simulink model "Forward_and_inverse_Both"  (R2024b)
settings: Solver=VariableStepAuto  StartTime=0.0  StopTime=7  MaxStep=0.005  RelTol=1e-3
model workspace: external: MATLAB File D:\OneDrive - itc.edu.kh\V4_robot_arm\Import_arm6\Test_Assembly_DataFile.m (data not in the file)
values from neighbouring files (symbols this model uses):
  Reach_max = max(REACH_MAX)    [Workspace_sample.m]
  Reach_min = max(REACH_MIN)    [Workspace_sample.m]
undefined symbols (not defined in the file or in its folder): DiscIntNeverNeededParam, initialPose, maxAngularAcc, maxAngularVel, maxLinearAcc, maxLinearVel, poseTol, smiData, Ts, wps1, X, Y, Z
libraries: sm_lib x140, nesl_utility x52, stmnucleolib x12, simulink x4, vrlib x2, vexcommonlib x2, robotcorelib x2
(part 1 of 6)
settings Model: PacingRate=0.010000  Creator=ASUS  LastModifiedBy=Bro_Chhay
settings OptimizationCC: ReuseModelBlockBuffer=off
settings DebuggingCC: AlgebraicLoopMsg=none  ArtificialAlgebraicLoopMsg=none  InheritedTsInSrcMsg=none
settings RTWCC: GPUComputeCapability=3.5
settings ExplorerConfigSet: InternalSimMechanicsExplorerSettings="<ExplorerConfiguration><canonicalview>default</canonicalview><AnimationSetting><BasePlaybackSpeed>1.0</BasePlaybackSpeed><PlaybackSpeedFactor>1.0</PlaybackSpeedFactor></AnimationSetting><TilePanel><TileInfo><Tiles Columns=\"2\" Count=\"4\" Rows=\"2\"><Column Weight=\"0.5\"/><Column Weight=\"0.5\"/><Row Weight=\"0.5\"/><Row Weight=\"0.5\"/><Tile Height=\"1\" Width=\"1\" X=\"0\" Y=\"0\"/><Tile Height=\"1\" Width=\"1\" X=\"0\" Y=\"1\"/><Tile Height=\"1\" Width=\"1\" X=\"1\" Y=\"0\"/><Tile Height=\"1\" Width=\"1\" X=\"1\" Y=\"1\"/></Tiles></TileInfo><SceneInfo><SceneViewer><BGColor><R>0.800000011920928955</R><G>0.800000011920928955</G><B>0.800000011920928955</B></BGColor><Camera><DoPerspective>off</DoPerspective><Position><X>112.042507163595758</X><Y>-707.89174178180906</Y><Z>378.03229364224967</Z></Position><Center><X>112.042507163595758</X><Y>2.99999040381362647</Y><Z>378.03229364224967</Z></Center><Up><X>0</X><Y>-0</Y><Z>1</Z></Up><ViewLimDist>1</ViewLimDist><YLim>389.373256225585919</YLim><XLim>528.596833306246026</XLim></Camera></SceneViewer><SceneViewer><BGColor><R>0.800000011920928955</R><G>0.800000011920928955</G><B>0.800000011920928955</B></BGColor><Camera><DoPerspective>off</DoPerspective><Position><X>112.042507163595758</X><Y>2.9999928452198219</Y><Z>1115.74949456857576</Z></Position><Center><X>112.042507163595758</X><Y>2.9999928452198219</Y><Z>378.032280824866803</Z></Center><Up><X>0</X><Y>1</Y><Z>-0</Z></Up><ViewLimDist>1</ViewLimDist><YLim>238.200927829742426</YLim><XLim>323.371608420028224</XLim></Camera></SceneViewer><SceneViewer><BGColor><R>0.800000011920928955</R><G>0.800000011920928955</G><B>0.800000011920928955</B></BGColor><Camera><DoPerspective>off</DoPerspective><Position><X>811.571529227276983</X><Y>2.9999928452198219</Y><Z>378.03229364224967</Z></Position><Center><X>112.042497397970806</X><Y>2.9999928452198219</Y><Z>378.03229364224967</Z></Center><Up><X>-0</X><Y>0</Y><Z>1</Z></Up><ViewLimDist>1</ViewLimDist><YLim>389.373256225585919</YLim><XLim>528.596833306246026</XLim></Camera></SceneViewer><SceneViewer><BGColor><R>0.800000011920928955</R><G>0.800000011920928955</G><B>0.800000011920928955</B></BGColor><Camera><DoPerspective>off</DoPerspective><Position><X>445.528454458655347</X><Y>-387.561072008495501</Y><Z>798.922774330656011</Z></Position><Center><X>57.2226628192288871</X><Y>0.744719630931172105</Y><Z>410.616982691205294</Z></Center><Up><X>-0.408248290463863073</X><Y>0.408248290463863073</Y><Z>0.816496580927726145</Z></Up><ViewLimDist>1</ViewLimDist><YLim>413.2447509765625</YLim><XLim>561.003775308298486</XLim></Camera></SceneViewer></SceneInfo></TilePanel><MechEditorPanel><Cameras/><GfxPanelCameraMap/><VideoCreator><PlaybackSpeedRatio>1.0</PlaybackSpeedRatio><FrameRate>60</FrameRate><VideoFormat>MPEG-4</VideoFormat><FrameSize>[1920 1080]</FrameSize></VideoCreator></MechEditorPanel></ExplorerConfiguration>"

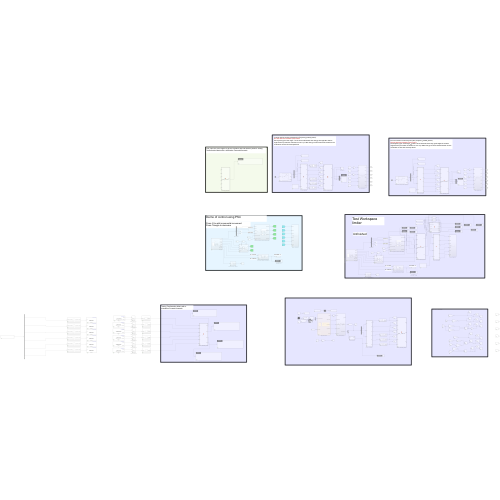
[thumbnail: Simulink's stored preview of the top-level diagram]
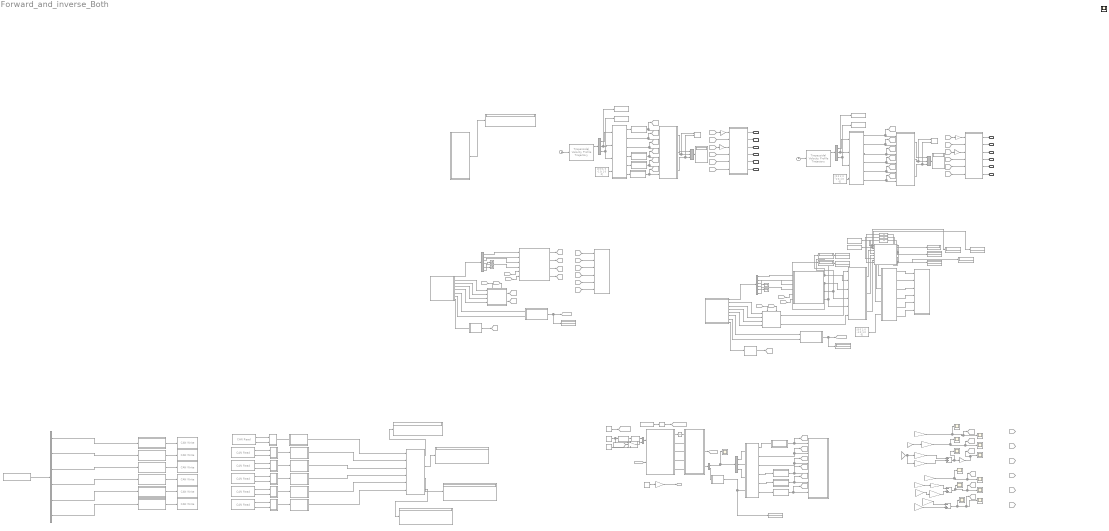
== system Forward_and_inverse_Both ==
  note: First we need to run the trajectory file (Trajectory_matlab_test.m).
      | Give the desired orientation (3x3) matrix.
      | The trajectory give Joint angle $\theta$ to the inverse kinematic then they go throught the relative angle block to prevention of theata run over 2 pi. After that, go to the forward kinematic for the verification as also the simscape block.
  note: cheak after Tranmission
  note: First, input the Joint angles to get the orietaion and end-effector position.Testing Tranformation Matrix with a simlulation Forward Kinematic.
  note: Testing Tranformation Matrix with a simlulation Forward Kinematic
  note: First we need to run the trajectory file (Trajectory_matlab_test.m).
      | Give the desired orientation (3x3) matrix.
      | The trajectory give Joint angle $\theta$ to the inverse kinematic then they go throught the relative angle block to prevention of theata run over 2 pi. After that, go to the forward kinematic for the verification as also the simscape block.
  note: Tri = decrease
  note: O = increase
  note: Initial Delta = 0
  note: Tri = decrease
  note: JoyStick Right
  note: JoyStick Left
  note: O = increase
  note: JoyStick Right
  note: Unfinished
  note: Demo of control using PS4
  note: JoyStick Left
  note: Test Workspace limiter
  note: Press O to add incremental movement
      | Press Triangle to decrease
  note: Initial Delta = 0
  0 ≤ Delta ≤ 0.1 Increment = 0.025 : Display  Commented=on
  0 ≤ Delta ≤ 0.1 Increment = 0.1 : Display  Commented=on
  {1..6} (6 alike) : stmnucleolib/CAN Read  Commented=on  CANModule=1  Identifier=Standard (11-bit identifier)  MsgId=246  MsgLen=8  RemoteFrame=off  OutputStatus=on  SampleTime=-1
      settings: LibrarySourceBlock=stmnucleoh7lib/CAN Read  DataFormat=Raw Data
  6 DOF robot arm : Subsystem  Commented=on
  6 DOF robot arm2 : Subsystem  Commented=on
  Add1 : Sum  Commented=on
  Add2 : Sum  Commented=on  Inputs=-+
  Add3 : Sum  Commented=on  Inputs=-+
  CAN Write : stmnucleolib/CAN Write  Commented=on  CANModule=0  Identifier=Standard (11-bit identifier)  MsgId=1  MsgLen=8  RemoteFrame=off  OutputStatus=off
      settings: LibrarySourceBlock=stmnucleoh7lib/CAN Write  DataFormat=Raw Data
  CAN Write1 : stmnucleolib/CAN Write  Commented=on  CANModule=0  Identifier=Standard (11-bit identifier)  MsgId=2  MsgLen=8  RemoteFrame=off  OutputStatus=off
      settings: LibrarySourceBlock=stmnucleoh7lib/CAN Write  DataFormat=Raw Data
  CAN Write2 : stmnucleolib/CAN Write  Commented=on  CANModule=0  Identifier=Standard (11-bit identifier)  MsgId=3  MsgLen=8  RemoteFrame=off  OutputStatus=off
      settings: LibrarySourceBlock=stmnucleoh7lib/CAN Write  DataFormat=Raw Data
  CAN Write3 : stmnucleolib/CAN Write  Commented=on  CANModule=0  Identifier=Standard (11-bit identifier)  MsgId=4  MsgLen=8  RemoteFrame=off  OutputStatus=off
      settings: LibrarySourceBlock=stmnucleoh7lib/CAN Write  DataFormat=Raw Data
  CAN Write4 : stmnucleolib/CAN Write  Commented=on  CANModule=0  Identifier=Standard (11-bit identifier)  MsgId=5  MsgLen=8  RemoteFrame=off  OutputStatus=off
      settings: LibrarySourceBlock=stmnucleoh7lib/CAN Write  DataFormat=Raw Data
  CAN Write5 : stmnucleolib/CAN Write  Commented=on  CANModule=0  Identifier=Standard (11-bit identifier)  MsgId=6  MsgLen=8  RemoteFrame=off  OutputStatus=off
      settings: LibrarySourceBlock=stmnucleoh7lib/CAN Write  DataFormat=Raw Data
  Clock : Clock  Commented=on
  Clock1 : Clock  Commented=on
  Constant1 : Constant  Commented=on
  Constant11 : Constant  Commented=on  Value=[0 0 1; 0 -1 0; 1 0 0]
  Constant12 : Constant  Commented=on  Value=Reach_max
  Constant13 : Constant  Commented=on  Value=0
  Constant14 : Constant  Commented=on  Value=initialPose
  Constant15 : Constant  Commented=on  Value=Reach_min
  Constant2 : Constant  Commented=on  Value=[0 0 0 0 0 0]
  Constant3 : Constant  Commented=on  Value=[0 0 1; 0 -1 0; 1 0 0]
  Constant4 : Constant  Commented=on  Value=[0 0 1; 0 -1 0; 1 0 0]
  Counter Free-Running : simulink/Sources/Counter Free-Running  Commented=on  NumBits=16  tsamp=-1
  Data Transform1 : Subsystem  Commented=on
  Data Transform2 : Subsystem  Commented=on
  Data Transform3 : Subsystem  Commented=on
  Data Transform4 : Subsystem  Commented=on
  Data Transform5 : Subsystem  Commented=on
  Data Transform6 : Subsystem  Commented=on
  Data Type Conversion : DataTypeConversion  Commented=on  OutDataTypeStr=double  SaturateOnIntegerOverflow=off  RndMeth=Floor
  Demux2 : Demux  Commented=on  Outputs=3
  Demux3 : Demux  Commented=on  Outputs=[3,1]
  Demux5 : Demux  Commented=on  Outputs=3
  Demux6 : Demux  Commented=on  Outputs=3
  Demux8 : Demux  Commented=on  Outputs=6
  Detect Increase : simulink/Logic and Bit Operations/Detect Increase  Commented=on  vinit=0.0  OutDataTypeStr=boolean
  Display{,1..14,17..19} (18 alike) : Display  Commented=on
  Flip the state of a button : Subsystem  Commented=on
  Flip the state of a button1 : Subsystem  Commented=on
  Forward_Kinematic : MATLAB Function  Commented=on  TreatAsAtomicUnit=on
  Forward_Kinematic_Good1 : MATLAB Function  Commented=on  TreatAsAtomicUnit=on
  Forward_Kinematic_Good2 : MATLAB Function  Commented=on  TreatAsAtomicUnit=on
  Forward_Kinematic_Good3 : MATLAB Function  Commented=on  TreatAsAtomicUnit=on
  Forward_Kinematic_Good4 : MATLAB Function  Commented=on  TreatAsAtomicUnit=on
  Forward_Kinematic_Good5 : MATLAB Function  Commented=on  TreatAsAtomicUnit=on
  From{,22..23,38} (4 alike) : From  Commented=on  GotoTag=n
  From1 : From  Commented=on  GotoTag=genPose
  From{10,13,28,36} (4 alike) : From  Commented=on  GotoTag=J5
  From{11,14,29,39} (4 alike) : From  Commented=on  GotoTag=J6
  From{9,12,27,35} (4 alike) : From  Commented=on  GotoTag=J4
  From{15,21,30,37} (4 alike) : From  Commented=on  GotoTag=Delta
  From{2,6,24,32} (4 alike) : From  Commented=on  GotoTag=J1
  From{3,7,25,33} (4 alike) : From  Commented=on  GotoTag=J2
  From{4,8,26,34} (4 alike) : From  Commented=on  GotoTag=J3
  From5 : From  Commented=on  GotoTag=simulation
  Gain{1..2,4,9} (4 alike) : Gain  Commented=on  Gain=32/30
  Gain{10,12,14,16..19} (7 alike) : Gain  Commented=on  Gain=-1
  Gain11 : Gain  Commented=on  Gain=25/15
  Gain13 : Gain  Commented=on  Gain=25/15
  Gain15 : Gain  Commented=on  Gain=Ts  OutDataTypeStr=double
  Gain3 : Gain  Commented=on  Gain=50/16
  Gain5 : Gain  Commented=on  Gain=72/22
  Gain6 : Gain  Commented=on  Gain=48/22
  Gain7 : Gain  Commented=on  Gain=50/36  OutDataTypeStr=Inherit: Same as input
  Gain8 : Gain  Commented=on  Gain=48/22
  Goto{,16,22,38} (4 alike) : Goto  Commented=on  GotoTag=J1
  Goto{1,17,23,37} (4 alike) : Goto  Commented=on  GotoTag=J2
  Goto10 : Goto  Commented=on  GotoTag=q5
  Goto11 : Goto  Commented=on  GotoTag=q6
  Goto12 : Goto  Commented=on  GotoTag=simulation
  Goto13 : Goto  Commented=on  GotoTag=genPose
  Goto14 : Goto  Commented=on  GotoTag=initialPose  TagVisibility=global
  Goto15 : Goto  Commented=on  GotoTag=t  TagVisibility=global
  Goto{2,18,24,39} (4 alike) : Goto  Commented=on  GotoTag=J3
  Goto{3,19,25,40} (4 alike) : Goto  Commented=on  GotoTag=J4
  Goto{4,20,26,41} (4 alike) : Goto  Commented=on  GotoTag=J5
  Goto{5,21,27,43} (4 alike) : Goto  Commented=on  GotoTag=J6
  Goto28 : Goto  Commented=on  GotoTag=Delta
  Goto34 : Goto  Commented=on  GotoTag=n
  Goto36 : Goto  Commented=on  GotoTag=Delta
  Goto42 : Goto  Commented=on  GotoTag=n
  Goto6 : Goto  Commented=on  GotoTag=q1
  Goto7 : Goto  Commented=on  GotoTag=q2
  Goto8 : Goto  Commented=on  GotoTag=q3
  Goto9 : Goto  Commented=on  GotoTag=q4
  Inverse Kinematic : MATLAB Function  Commented=on  TreatAsAtomicUnit=on
  Inverse Kinematic1 : MATLAB Function  Commented=on  TreatAsAtomicUnit=on
  Inverse Kinematic2 : MATLAB Function  Commented=on  TreatAsAtomicUnit=on
  Inverse Kinematic4 : MATLAB Function  Commented=on  TreatAsAtomicUnit=on
  MATLAB Function : MATLAB Function  Commented=on  TreatAsAtomicUnit=on
  Mux : Mux  Commented=on  Inputs=3
  Mux1 : Mux  Commented=on  Inputs=3
  Mux3 : Mux  Commented=on  Inputs=2
  PS4 Demux : Demux  Commented=on  Outputs=6
  PS4 Demux1 : Demux  Commented=on  Outputs=6
  Pulse Generator : DiscretePulseGenerator  Commented=on  PulseType=Time based  Period=30  PulseWidth=5  PhaseDelay=5
  Reshape : Reshape  Commented=on  OutputDimensionality=Column vector (2-D)
  Rotation Matrix : MATLAB Function  Commented=on  TreatAsAtomicUnit=on
  Scope{1,3..14} (13 alike) : Scope  Commented=on
  "Set Delta for the joint movement more Delta, faster the movement" : Subsystem  Commented=on
  "Set Delta for the joint movement more Delta, faster the movement1" : Subsystem  Commented=on
  Set Joint position to where it were left off : Subsystem  Commented=on
  Set Joint position to where it were left off1 : Subsystem  Commented=on
  Simscape Robot1 : Subsystem  Commented=on
  Simscape Robot2 : Subsystem  Commented=on
  Subsystem : Subsystem  Commented=on
      settings: PortSchema="{\"entries\":[{\"content\":{\"sides\":[{\"content\":{\"connectorIds\":[\"In1\",\"In2\",\"In3\",\"In4\"]},\"type\":\"ConnectorPlacement.EquallySpacedRectSide\",\"uuid\":\"934df258-a69f-45fc-920e-d96d4c7e69c4\"},{\"content\":{\"connectorIds\":[\"Out1\",\"Out2\"],\"side\":\"RIGHT\"},\"type\":\"ConnectorPlacement.EquallySpacedRectSide\",\"uuid\":\"4248c0a4-0efa-4e68-894f-9df7c5b1e3ab\"},{\"content\":{\"connectorIds\":[\"In5\",\"In6\"],\"side\":\"TOP\"},\"type\":\"ConnectorPlacement.EquallySpacedRectSide\",\"uuid\":\"db1bee13-57d6-4361-8657-1365417e1e26\"}]},\"type\":\"ConnectorPlacement.EquallySpacedConnector\",\"uuid\":\"c32f6b1b-3465-4573-ab20-ef0ae83e0fed\"}],\"packageUris\":[\"http://schema.mathworks.com/mf0/Connector/R2020b\"],\"version\":\"1.0\"}"
  Subsystem1 : Subsystem  Commented=on
  Subsystem10 : Subsystem  Commented=on
  Subsystem11 : Subsystem  Commented=on
  Subsystem12 : Subsystem  Commented=on
  Subsystem13 : Subsystem  Commented=on
  Subsystem14 : Subsystem  Commented=on
  Subsystem15 : Subsystem  Commented=on
  Subsystem16 : Subsystem  Commented=on
  Subsystem17 : Subsystem  Commented=on
  Subsystem18 : Subsystem  Commented=on
  Subsystem19 : Subsystem  Commented=on
  Subsystem2 : Subsystem  Commented=on
  Subsystem20 : Subsystem  Commented=on
      settings: PortSchema="{\"entries\":[{\"content\":{\"sides\":[{\"content\":{\"connectorIds\":[\"In1\",\"In2\",\"In3\",\"In4\"]},\"type\":\"ConnectorPlacement.EquallySpacedRectSide\",\"uuid\":\"934df258-a69f-45fc-920e-d96d4c7e69c4\"},{\"content\":{\"connectorIds\":[\"Out1\",\"Out2\"],\"side\":\"RIGHT\"},\"type\":\"ConnectorPlacement.EquallySpacedRectSide\",\"uuid\":\"4248c0a4-0efa-4e68-894f-9df7c5b1e3ab\"},{\"content\":{\"connectorIds\":[\"In5\",\"In6\"],\"side\":\"TOP\"},\"type\":\"ConnectorPlacement.EquallySpacedRectSide\",\"uuid\":\"db1bee13-57d6-4361-8657-1365417e1e26\"}]},\"type\":\"ConnectorPlacement.EquallySpacedConnector\",\"uuid\":\"c32f6b1b-3465-4573-ab20-ef0ae83e0fed\"}],\"packageUris\":[\"http://schema.mathworks.com/mf0/Connector/R2020b\"],\"version\":\"1.0\"}"
  Subsystem21 : Subsystem  Commented=on
  Subsystem24 : Subsystem  Commented=on
  Subsystem25 : Subsystem  Commented=on
  Subsystem3 : Subsystem  Commented=on
  Subsystem4 : Subsystem  Commented=on
  Subsystem5 : Subsystem  Commented=on
  Subsystem6 : Subsystem  Commented=on
  Subsystem7 : Subsystem  Commented=on
  Subsystem8 : Subsystem  Commented=on
  Subsystem9 : Subsystem  Commented=on
  Switch4 : Switch  Commented=on  Criteria=u2 > Threshold  SaturateOnIntegerOverflow=off  InputSameDT=off
  Terminator{,1..3} (4 alike) : Terminator  Commented=on
  To Workspace : ToWorkspace  Commented=on  VariableName=Yin  SampleTime=-1
      settings: Save2DSignal=2-D array (concatenate along first dimension)
  To Workspace1 : ToWorkspace  Commented=on  VariableName=Zin1  SampleTime=-1
      settings: Save2DSignal=2-D array (concatenate along first dimension)
  To Workspace2 : ToWorkspace  Commented=on  VariableName=Yin1  SampleTime=-1
      settings: Save2DSignal=2-D array (concatenate along first dimension)
  To Workspace3 : ToWorkspace  Commented=on  VariableName=Zin  SampleTime=-1
      settings: Save2DSignal=2-D array (concatenate along first dimension)
  Trapezoidal Velocity Profile Trajectory : robotcorelib/Trapezoidal Velocity Profile Trajectory  Commented=on  WaypointSource=Internal  Waypoints=waypoints_6  NumParams=1  Parameter1=End Time  Parameter2=End Time  ParameterSource=Internal  PeakVelocity=[ 2; 2 ]  Acceleration=[ 1; 2 ]  EndTime=2  AccelTime=[ 1; 2 ]  SimulateUsing=Interpreted execution
  Trapezoidal Velocity Profile Trajectory1 : robotcorelib/Trapezoidal Velocity Profile Trajectory  Commented=on  WaypointSource=Internal  Waypoints=Way4  NumParams=1  Parameter1=End Time  Parameter2=End Time  ParameterSource=Internal  PeakVelocity=[ 2; 2 ]  Acceleration=[ 1; 2 ]  EndTime=2  AccelTime=[ 1; 2 ]  SimulateUsing=Interpreted execution
  Unit Delay{,1..3} (4 alike) : UnitDelay  Commented=on  SampleTime=-1  HasFrameUpgradeWarning=on
  Waypoint Planner : Stateflow chart  Commented=on  TreatAsAtomicUnit=on
      settings: PortSchema="{\"entries\":[{\"content\":{\"sides\":[{\"content\":{\"connectorIds\":[\"In2\",\"In1\"]},\"type\":\"ConnectorPlacement.EquallySpacedRectSide\",\"uuid\":\"2f7816bf-e041-4d80-a35c-f5abf025ca4f\"},{\"content\":{\"connectorIds\":[\"Out5\",\"Out1\",\"Out2\",\"Out3\",\"Out4\"],\"side\":\"RIGHT\"},\"type\":\"ConnectorPlacement.EquallySpacedRectSide\",\"uuid\":\"030a9877-c717-421f-9736-0adf27f6f35f\"},{\"content\":{\"side\":\"TOP\"},\"type\":\"ConnectorPlacement.EquallySpacedRectSide\",\"uuid\":\"ba023d22-bb45-4b84-a72f-1110f01393be\"}]},\"type\":\"ConnectorPlacement.EquallySpacedConnector\",\"uuid\":\"d2a85391-dfa2-4741-8917-4ca0c8ef44a5\"}],\"packageUris\":[\"http://schema.mathworks.com/mf0/Connector/R2020b\"],\"version\":\"1.0\"}"
  Waypoint Trajectory : Subsystem  Commented=on
  XY Graph1 : Record  Commented=on  VariableName=recordout2  RecordToWorkspace=on  FileSettingsInternal="{\"entries\":[{\"content\":{\"excelSettings\":{\"content\":{},\"type\":\"Streamout.ExcelSettings\"}},\"type\":\"Streamout.FileSettingStorage\",\"uuid\":\"\"}],\"packageUris\":[\"http:\\/\\/schema.mathworks.com\\/mf0\\/streamout_blocks\\/R2020a\"],\"version\":\"1.0\"}"  Layout=[1 1]  SignalsInternal="{\"entries\":[{\"content\":{},\"type\":\"RecordBlkView.InputSignals\",\"uuid\":\"\"}],\"packageUris\":[\"http:\\/\\/schema.mathworks.com\\/mf0\\/streamout_blocks\\/R2020a\"],\"version\":\"1.0\"}"  VisualizationBindings="{\"xyplotplugin\":{\"info\":[{\"series\":[],\"subplotID\":1}]}}"  CompatibilityTag=XY
  XY Graph2 : Record  Commented=on  VariableName=recordout2  RecordToWorkspace=on  FileSettingsInternal="{\"entries\":[{\"content\":{\"excelSettings\":{\"content\":{},\"type\":\"Streamout.ExcelSettings\"}},\"type\":\"Streamout.FileSettingStorage\",\"uuid\":\"\"}],\"packageUris\":[\"http:\\/\\/schema.mathworks.com\\/mf0\\/streamout_blocks\\/R2020a\"],\"version\":\"1.0\"}"  Layout=[1 1]  SignalsInternal="{\"entries\":[{\"content\":{\"signals\":[{\"content\":{\"blockPath\":[],\"dimensions\":[1],\"domain\":\"\",\"lineColor\":\"#a2142f\",\"plots\":[ 1 ],\"port\":1,\"signalID\":1,\"signalName\":\"Forward_Kinematic_Good4:2\"},\"type\":\"RecordBlkView.Signal\",\"uuid\":\"\"},{\"content\":{\"blockPath\":[],\"dimensions\":[1],\"domain\":\"\",\"lineColor\":\"#139fff\",\"plots\":[ 1 ],\"port\":2,\"signalID\":2,\"signalName\":\"Forward_Kinematic_Good4:3\"},\"type\":\"RecordBlkView.Signal\",\"uuid\":\"\"}]},\"type\":\"RecordBlkView.InputSignals\",\"uuid\":\"\"}],\"packageUris\":[\"http:\\/\\/schema.mathworks.com\\/mf0\\/streamout_blocks\\/R2020a\"],\"version\":\"1.0\"}"  VisualizationBindings="{\"xyplotplugin\":{\"info\":[{\"series\":[{\"bindingParametersList\":[{\"parameter\":\"X-Axis\",\"signalID\":1,\"signalName\":\"Forward_Kinematic_Good4:2\"},{\"parameter\":\"Y-Axis\",\"signalID\":2,\"signalName\":\"Forward_Kinematic_Good4:3\"}],\"seriesID\":0}],\"subplotID\":1}]}}"  CompatibilityTag=XY
  Output : Outport
  Output1 : Outport  Port=2
  Output2 : Outport  Port=3
  Output3 : Outport  Port=4
  Output4 : Outport  Port=5
  Output5 : Outport  Port=6
  Output6 : Outport  Port=7
  Output7 : Outport  Port=8
  Output8 : Outport  Port=9
  Output9 : Outport  Port=10
  Output10 : Outport  Port=11
  Output11 : Outport  Port=12
  Scope2 : Scope
  wires:
  Forward_Kinematic_Good2/4(R36) -> Display18/1
  Forward_Kinematic_Good2/3(R03) -> Display17/1
  Forward_Kinematic_Good2/2(R06) -> Display10/1
  Constant2/1 -> Demux8/1
  Forward_Kinematic_Good2/1(A06) -> Display19/1
  Demux8/3 -> Subsystem2/1(Desired Position)
  Subsystem1/1(Output to CAN) -> CAN Write1/1
  Demux8/1 -> Subsystem4/1(Desired Position)
  Subsystem5/1(Output to CAN) -> CAN Write4/1
  Subsystem6/1(Output to CAN) -> CAN Write5/1
  Demux8/5 -> Subsystem5/1(Desired Position)
  Demux8/6 -> Subsystem6/1(Desired Position)
  Subsystem2/1(Output to CAN) -> CAN Write2/1
  Subsystem4/1(Output to CAN) -> CAN Write/1
  Demux8/2 -> Subsystem1/1(Desired Position)
  Demux8/4 -> Subsystem3/1(Desired Position)
  Subsystem3/1(Output to CAN) -> CAN Write3/1
  Data Transform2/1(Data_T) -> Subsystem8/1(data)
  Subsystem7/1(position) -> Forward_Kinematic_Good2/1(th1)
  Data Transform3/1(Data_T) -> Subsystem9/1(data)
  Subsystem11/1(position) -> Forward_Kinematic_Good2/5(th5)
  Subsystem12/1(position) -> Forward_Kinematic_Good2/6(th6)
  Subsystem10/1(position) -> Forward_Kinematic_Good2/4(th4)
  Data Transform5/1(Data_T) -> Subsystem11/1(data)
  Subsystem8/1(position) -> Forward_Kinematic_Good2/2(th2)
  1/2 -> Data Transform2/2(In2)
  6/1 -> Data Transform6/1(In1)
  6/2 -> Data Transform6/2(In2)
  2/2 -> Data Transform3/2(In2)
  Data Transform1/1(Data_T) -> Subsystem7/1(data)
  5/1 -> Data Transform5/1(In1)
  4/2 -> Data Transform4/2(In2)
  Data Transform6/1(Data_T) -> Subsystem12/1(data)
  3/2 -> Data Transform1/2(In2)
  Data Transform4/1(Data_T) -> Subsystem10/1(data)
  2/1 -> Data Transform3/1(In1)
  3/1 -> Data Transform1/1(In1)
  4/1 -> Data Transform4/1(In1)
  1/1 -> Data Transform2/1(In1)
  5/2 -> Data Transform5/2(In2)
  Subsystem9/1(position) -> Forward_Kinematic_Good2/3(th3)
  Gain3/1 -> Scope6/1, Scope12/1, Goto9/1  "J4"
  Gain5/1 -> Scope10/1, Goto7/1, Scope4/1  "J2"
  Gain1/1 -> Add2/1
  Gain8/1 -> Add1/2
  Add1/1 -> Gain12/1, Scope5/1  "J3"
  Gain4/1 -> Add3/2
  Gain6/1 -> Add1/1
  Gain13/1 -> Gain9/1
  Gain7/1 -> Scope3/1, Scope9/1, Goto6/1  "J1"
  Add2/1 -> Scope7/1, Scope13/1, Goto10/1  "J5"
  Gain11/1 -> Gain1/1
  Add3/1 -> Scope8/1, Scope14/1, Goto11/1  "J6"
  Gain9/1 -> Add2/2
  Trapezoidal Velocity Profile Trajectory/1 -> Demux6/1
  Gain12/1 -> Scope11/1, Goto8/1
  Gain2/1 -> Add3/1
  Gain10/1 -> Gain5/1
  Gain14/1 -> Gain8/1, Gain6/1
  Constant13/1 -> Switch4/3
  Waypoint Trajectory/2(genPose) -> Goto13/1
  Demux3/2 -> Rotation Matrix/1(roll)
  Waypoint Planner/3(targetPose) -> Waypoint Trajectory/4(targetPose)
  Waypoint Trajectory/3(filteredPose) -> Demux3/1
  Switch4/1 -> Mux3/2
  Mux3/1 -> Waypoint Planner/2(semiAutoButton)
  Waypoint Planner/1(departTime) -> Waypoint Trajectory/2(departTime)
  From1/1 -> Waypoint Planner/1(genPose)
  Detect Increase/1 -> Data Type Conversion/1
  Pulse Generator/1 -> Switch4/1, Detect Increase/1
  Unit Delay/1 -> Waypoint Trajectory/1(mode)
  Waypoint Planner/4(maxVel) -> Waypoint Trajectory/5(maxVel)
  Demux3/1 -> Demux5/1, Scope1/1
  Counter Free-Running/1 -> Gain15/1
  Reshape/1 -> Goto14/1
  Rotation Matrix/1(R06) -> Display/1, Inverse Kinematic1/4(R06)
  Waypoint Planner/2(departPose) -> Waypoint Trajectory/3(departPose)
  Gain15/1 -> Goto15/1
  Constant1/1 -> Goto12/1
  Data Type Conversion/1 -> Mux3/1
  Constant14/1 -> Reshape/1
  From5/1 -> Switch4/2
  Waypoint Planner/5(mode) -> Unit Delay/1
  Subsystem16/1(angle) -> Forward_Kinematic_Good3/5(th5), Goto4/1
  Subsystem17/1(angle) -> Forward_Kinematic_Good3/6(th6), Goto5/1
  Inverse Kinematic1/4(q4) -> Subsystem15/1(q1)
  Inverse Kinematic1/1(q1) -> Subsystem13/1(q1)
  Inverse Kinematic1/6(q6) -> Subsystem17/1(q1)  "q6"
  Inverse Kinematic1/3(q3) -> Goto2/1, Forward_Kinematic_Good3/3(th3)  "q3"
  Inverse Kinematic1/5(q5) -> Subsystem16/1(q1)
  Subsystem13/1(angle) -> Forward_Kinematic_Good3/1(th1), Goto/1
  Inverse Kinematic1/2(q2) -> Forward_Kinematic_Good3/2(th2), Goto1/1  "q2"
  Subsystem15/1(angle) -> Forward_Kinematic_Good3/4(th4), Goto3/1
  Demux5/1 -> Inverse Kinematic1/1(Px)
  Demux5/2 -> Inverse Kinematic1/2(Py)
  Demux5/3 -> Inverse Kinematic1/3(Pz)
  Subsystem14/1(angle) -> Forward_Kinematic_Good1/1(th1), Goto16/1
  Inverse Kinematic/4(q4) -> Subsystem18/1(q1)
  Demux6/2 -> To Workspace/1, Inverse Kinematic/2(Py)
  Inverse Kinematic/3(q3) -> Forward_Kinematic_Good1/3(th3), Goto18/1  "q3"
  Demux6/3 -> To Workspace1/1, Inverse Kinematic/3(Pz)
  Subsystem25/1(angle) -> Forward_Kinematic_Good1/6(th6), Goto21/1
  Inverse Kinematic/2(q2) -> Forward_Kinematic_Good1/2(th2), Goto17/1  "q2"
  Inverse Kinematic/6(q6) -> Subsystem25/1(q1)  "q6"
  Inverse Kinematic/5(q5) -> Subsystem24/1(q1)
  Inverse Kinematic/1(q1) -> Subsystem14/1(q1)
  Demux6/1 -> Inverse Kinematic/1(Px)
  Subsystem18/1(angle) -> Forward_Kinematic_Good1/4(th4), Goto19/1
  Constant3/1 -> Inverse Kinematic/4(R06)
  Subsystem24/1(angle) -> Forward_Kinematic_Good1/5(th5), Goto20/1
  Forward_Kinematic_Good1/2(Py) -> XY Graph1/1, Mux/2
  Forward_Kinematic_Good1/3(Pz) -> Mux/3, XY Graph1/2
  Forward_Kinematic_Good1/1(Px) -> Mux/1
  Mux/1 -> Display2/1
  Clock/1 -> Trapezoidal Velocity Profile Trajectory/1
  From24/1 -> Gain18/1
  From25/1 -> Simscape Robot1/2(q2)
  Gain16/1 -> Simscape Robot1/3(q3)
  Gain18/1 -> Simscape Robot1/1(q1)
  From27/1 -> Simscape Robot1/4(q4)
  From26/1 -> Gain16/1
  From29/1 -> Simscape Robot1/6(q6)
  From28/1 -> Simscape Robot1/5(q5)
  Simscape Robot1/1(qm1) -> Output/1
  Simscape Robot1/2(qm2) -> Output1/1
  Simscape Robot1/3(qm3) -> Output2/1
  Simscape Robot1/4(qm4) -> Output3/1
  Simscape Robot1/5(qm5) -> Output4/1
  Simscape Robot1/6(qm6) -> Output5/1
  Simscape Robot2/2(qm2) -> Output7/1
  Simscape Robot2/3(qm3) -> Output8/1
  Simscape Robot2/6(qm6) -> Output11/1
  Simscape Robot2/5(qm5) -> Output10/1
  Gain19/1 -> Simscape Robot2/1(q1)
  From3/1 -> Simscape Robot2/2(q2)
  Simscape Robot2/4(qm4) -> Output9/1
  From13/1 -> Simscape Robot2/5(q5)
  Inverse Kinematic2/4(q4) -> Forward_Kinematic_Good4/4(th4), Goto25/1
  Inverse Kinematic2/3(q3) -> Goto24/1, Forward_Kinematic_Good4/3(th3)  "q3"
  Demux2/2 -> To Workspace2/1, Inverse Kinematic2/2(Py)
  Forward_Kinematic_Good4/2(Py) -> XY Graph2/1, Mux1/2
  From14/1 -> Simscape Robot2/6(q6)
  Forward_Kinematic_Good4/3(Pz) -> Mux1/3, XY Graph2/2
  Inverse Kinematic2/6(q6) -> Forward_Kinematic_Good4/6(th6), Goto27/1  "q6"
  Inverse Kinematic2/1(q1) -> Forward_Kinematic_Good4/1(th1), Goto22/1
  Inverse Kinematic2/5(q5) -> Forward_Kinematic_Good4/5(th5), Goto26/1
  Forward_Kinematic_Good4/1(Px) -> Mux1/1
  Clock1/1 -> Trapezoidal Velocity Profile Trajectory1/1
  Demux2/1 -> Inverse Kinematic2/1(Px)
  Constant4/1 -> Inverse Kinematic2/4(R06)
  Demux2/3 -> To Workspace3/1, Inverse Kinematic2/3(Pz)
  From2/1 -> Gain19/1
  Mux1/1 -> Display1/1
  Trapezoidal Velocity Profile Trajectory1/1 -> Demux2/1
  Inverse Kinematic2/2(q2) -> Forward_Kinematic_Good4/2(th2), Goto23/1  "q2"
  From4/1 -> Gain17/1
  Gain17/1 -> Simscape Robot2/3(q3)
  Simscape Robot2/1(qm1) -> Output6/1
  From12/1 -> Simscape Robot2/4(q4)
  Forward_Kinematic/1(A0_6) -> Display4/1
  From36/1 -> 6 DOF robot arm2/5(joint5)
  PS4 Demux1/3 -> Set Joint position to where it were left off1/3(pos2)
  Subsystem21/6(D8_left) -> "Set Delta for the joint movement more Delta, faster the movement1"/1(O)
  Set Joint position to where it were left off1/1(posfinal2) -> Goto37/1
  Subsystem21/1(Out1) -> PS4 Demux1/1
  From15/1 -> Set Joint position to where it were left off/5(pos incremental)
  From22/1 -> Subsystem/6(n)
  Constant15/1 -> Display8/1, MATLAB Function/1(Reach_min)
  Set Joint position to where it were left off1/4(posfinal5) -> Goto41/1
  Inverse Kinematic4/4(q4) -> 6 DOF robot arm/4(joint4)
  Subsystem19/7(D8_down) -> "Set Delta for the joint movement more Delta, faster the movement"/2(Tri)
  From23/1 -> Set Joint position to where it were left off1/6(coeff to set pos 0)
  MATLAB Function/1(x_out) -> Unit Delay2/1, Inverse Kinematic4/1(Px), Display3/1
  From37/1 -> Subsystem20/5(delta)
  Subsystem21/2(D5_up) -> Subsystem20/1(L1)
  Subsystem21/4(D_right) -> Subsystem20/3(Dpad R)
  PS4 Demux1/1 -> Set Joint position to where it were left off1/1(pos1)
  Subsystem19/8(D8_right) -> Flip the state of a button/1(X)
  From/1 -> Set Joint position to where it were left off/6(coeff to set pos 0)
  Subsystem21/3(D6_up) -> Subsystem20/2(R1)
  From21/1 -> Subsystem/5(delta)
  Flip the state of a button1/1(n_out) -> Goto42/1
  Subsystem21/8(D8_right) -> Flip the state of a button1/1(X)
  Subsystem19/1(Out1) -> PS4 Demux/1
  From39/1 -> 6 DOF robot arm2/6(joint6)
  PS4 Demux/1 -> Set Joint position to where it were left off/1(pos1)
  Set Joint position to where it were left off/2(posfinal3) -> Display12/1, Forward_Kinematic_Good5/3(th3)
  Subsystem19/5(D_left) -> Subsystem/4(Dpad L)
  Unit Delay2/1 -> MATLAB Function/4(x_error)
  From33/1 -> 6 DOF robot arm2/2(joint2)
  PS4 Demux1/6 -> Set Joint position to where it were left off1/4(pos4)
  Constant11/1 -> Inverse Kinematic4/4(R06)
  Inverse Kinematic4/6(q6) -> 6 DOF robot arm/6(joint6)  "q6"
  Forward_Kinematic_Good5/3(Pz) -> MATLAB Function/7(z)
  Set Joint position to where it were left off/1(posfinal2) -> Display11/1, Forward_Kinematic_Good5/2(th2)
  Subsystem20/2(J6) -> Goto43/1
  "Set Delta for the joint movement more Delta, faster the movement"/1(Output) -> 0 ≤ Delta ≤ 0.1 Increment = 0.025/1, Goto28/1
  PS4 Demux1/4 -> Terminator2/1
  Subsystem/2(J6) -> Forward_Kinematic_Good5/6(th6)
  Unit Delay1/1 -> MATLAB Function/6(y_error)
  Inverse Kinematic4/2(q2) -> 6 DOF robot arm/2(joint2)  "q2"
  Subsystem19/2(D5_up) -> Subsystem/1(L1)
  Subsystem21/5(D_left) -> Subsystem20/4(Dpad L)
  PS4 Demux/6 -> Set Joint position to where it were left off/4(pos4)
  PS4 Demux/2 -> Set Joint position to where it were left off/2(pos3)
  From34/1 -> 6 DOF robot arm2/3(joint3)
  Set Joint position to where it were left off1/3(posfinal4) -> Goto40/1
  "Set Delta for the joint movement more Delta, faster the movement1"/1(Output) -> 0 ≤ Delta ≤ 0.1 Increment = 0.1/1, Goto36/1
  From38/1 -> Subsystem20/6(n)
  Set Joint position to where it were left off/4(posfinal5) -> Display14/1, Forward_Kinematic_Good5/5(th5)
  From32/1 -> 6 DOF robot arm2/1(joint1)
  Set Joint position to where it were left off/3(posfinal4) -> Display13/1, Forward_Kinematic_Good5/4(th4)
  PS4 Demux1/2 -> Set Joint position to where it were left off1/2(pos3)
  Inverse Kinematic4/1(q1) -> 6 DOF robot arm/1(joint1)
  From35/1 -> 6 DOF robot arm2/4(joint4)
  Inverse Kinematic4/3(q3) -> 6 DOF robot arm/3(joint3)  "q3"
  Forward_Kinematic_Good5/2(Py) -> MATLAB Function/5(y)
  Subsystem21/7(D8_down) -> "Set Delta for the joint movement more Delta, faster the movement1"/2(Tri)
  Forward_Kinematic_Good5/1(Px) -> MATLAB Function/3(x)
  From30/1 -> Set Joint position to where it were left off1/5(pos incremental)
  Subsystem19/3(D6_up) -> Subsystem/2(R1)
  Flip the state of a button/1(n_out) -> Goto34/1
  Subsystem20/1(J1) -> Goto38/1
  Constant12/1 -> Display9/1, MATLAB Function/2(Reach_max)
  Subsystem19/6(D8_left) -> "Set Delta for the joint movement more Delta, faster the movement"/1(O)
  Subsystem19/4(D_right) -> Subsystem/3(Dpad R)
  PS4 Demux/4 -> Terminator/1
  PS4 Demux/3 -> Set Joint position to where it were left off/3(pos2)
  PS4 Demux1/5 -> Terminator3/1
  Subsystem/1(J1) -> Forward_Kinematic_Good5/1(th1)
  MATLAB Function/4(Out) -> Display7/1
  MATLAB Function/3(z_out) -> Display6/1, Unit Delay3/1, Inverse Kinematic4/3(Pz)
  Unit Delay3/1 -> MATLAB Function/8(z_error)
  MATLAB Function/2(y_out) -> Unit Delay1/1, Inverse Kinematic4/2(Py), Display5/1
  PS4 Demux/5 -> Terminator1/1
  Set Joint position to where it were left off1/2(posfinal3) -> Goto39/1
  Inverse Kinematic4/5(q5) -> 6 DOF robot arm/5(joint5)

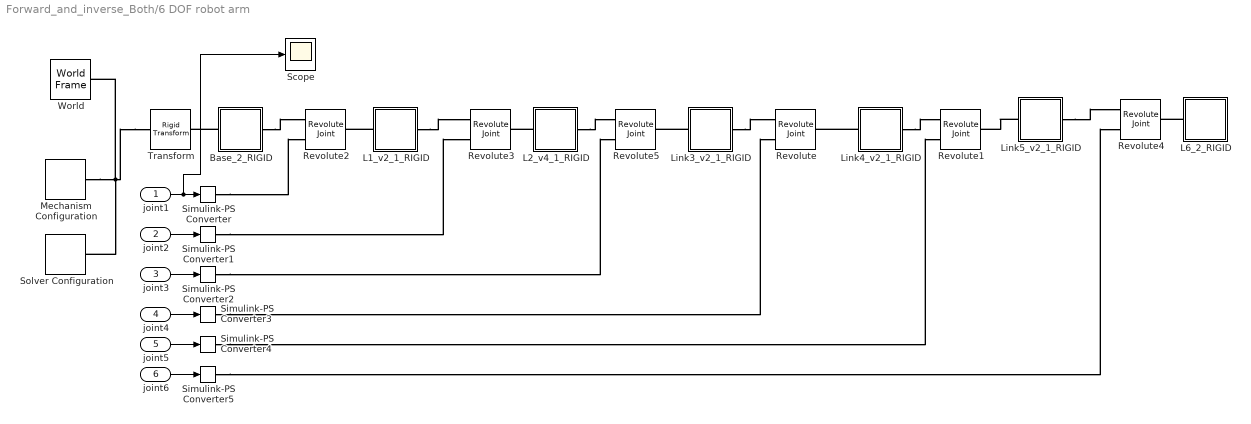
== system Forward_and_inverse_Both/6 DOF robot arm ==
  joint1 : Inport
  joint2 : Inport  Port=2
  joint3 : Inport  Port=3
  joint4 : Inport  Port=4
  joint5 : Inport  Port=5
  joint6 : Inport  Port=6
  Base_2_RIGID : Subsystem
  L1_v2_1_RIGID : Subsystem
  L2_v4_1_RIGID : Subsystem
  L6_2_RIGID : Subsystem
  Link3_v2_1_RIGID : Subsystem
  Link4_v2_1_RIGID : Subsystem
  Link5_v2_1_RIGID : Subsystem
  Mechanism Configuration : sm_lib/Utilities/Mechanism Configuration  UniformGravity=Constant  GravityVector=[0 0 -9.80665]  GravityVectorUnits=m/s^2  LinearizationDelta=0.001  JointModeTransitionNonlinearIterations=2
  Revolute : sm_lib/Joints/Revolute Joint  JointMode=Normal  CompositeWrenchDir=FollowerOnBase  CompositeWrenchFrame=BaseFrame  SenseConstraintForce=off  SenseConstraintTorque=off  SenseTotalForce=off  SenseTotalTorque=off  PositionTargetSpecify=off  PositionTargetPriority=Low  PositionTargetValue=smiData.RevoluteJoint(1).Rz.Pos  PositionTargetValueUnits=deg  VelocityTargetSpecify=off  VelocityTargetPriority=High  VelocityTargetValue=0  VelocityTargetValueUnits=deg/s  EquilibriumPosition=0  EquilibriumPositionUnits=deg  SpringStiffness=0  SpringStiffnessUnits=N*m/deg  DampingCoefficient=0  DampingCoefficientUnits=N*m/(deg/s)  LowerLimitSpecify=off  LowerLimitBound=-90  LowerLimitBoundUnits=deg  LowerLimitStiffness=1e4  LowerLimitStiffnessUnits=N*m/deg  LowerLimitDamping=10  LowerLimitDampingUnits=N*m/(deg/s)  LowerLimitTransitionRegionWidth=0.1  LowerLimitTransitionRegionWidthUnits=deg  UpperLimitSpecify=off  UpperLimitBound=90  UpperLimitBoundUnits=deg  UpperLimitStiffness=1e4  UpperLimitStiffnessUnits=N*m/deg  UpperLimitDamping=10  UpperLimitDampingUnits=N*m/(deg/s)  UpperLimitTransitionRegionWidth=0.1  UpperLimitTransitionRegionWidthUnits=deg  TorqueActuationMode=ComputedTorque  MotionActuationMode=InputMotion  SensePosition=off  SenseVelocity=off  SenseAcceleration=off  SenseTorqueForce=off  SenseLowerLimitTorqueForce=off  SenseUpperLimitTorqueForce=off
  Revolute1 : sm_lib/Joints/Revolute Joint  JointMode=Normal  CompositeWrenchDir=FollowerOnBase  CompositeWrenchFrame=BaseFrame  SenseConstraintForce=off  SenseConstraintTorque=off  SenseTotalForce=off  SenseTotalTorque=off  PositionTargetSpecify=off  PositionTargetPriority=Low  PositionTargetValue=smiData.RevoluteJoint(2).Rz.Pos  PositionTargetValueUnits=deg  VelocityTargetSpecify=off  VelocityTargetPriority=High  VelocityTargetValue=0  VelocityTargetValueUnits=deg/s  EquilibriumPosition=0  EquilibriumPositionUnits=deg  SpringStiffness=0  SpringStiffnessUnits=N*m/deg  DampingCoefficient=0  DampingCoefficientUnits=N*m/(deg/s)  LowerLimitSpecify=off  LowerLimitBound=-90  LowerLimitBoundUnits=deg  LowerLimitStiffness=1e4  LowerLimitStiffnessUnits=N*m/deg  LowerLimitDamping=10  LowerLimitDampingUnits=N*m/(deg/s)  LowerLimitTransitionRegionWidth=0.1  LowerLimitTransitionRegionWidthUnits=deg  UpperLimitSpecify=off  UpperLimitBound=90  UpperLimitBoundUnits=deg  UpperLimitStiffness=1e4  UpperLimitStiffnessUnits=N*m/deg  UpperLimitDamping=10  UpperLimitDampingUnits=N*m/(deg/s)  UpperLimitTransitionRegionWidth=0.1  UpperLimitTransitionRegionWidthUnits=deg  TorqueActuationMode=ComputedTorque  MotionActuationMode=InputMotion  SensePosition=off  SenseVelocity=off  SenseAcceleration=off  SenseTorqueForce=off  SenseLowerLimitTorqueForce=off  SenseUpperLimitTorqueForce=off
  Revolute2 : sm_lib/Joints/Revolute Joint  JointMode=Normal  CompositeWrenchDir=FollowerOnBase  CompositeWrenchFrame=BaseFrame  SenseConstraintForce=off  SenseConstraintTorque=off  SenseTotalForce=off  SenseTotalTorque=off  PositionTargetSpecify=off  PositionTargetPriority=Low  PositionTargetValue=smiData.RevoluteJoint(3).Rz.Pos  PositionTargetValueUnits=deg  VelocityTargetSpecify=off  VelocityTargetPriority=High  VelocityTargetValue=0  VelocityTargetValueUnits=deg/s  EquilibriumPosition=0  EquilibriumPositionUnits=deg  SpringStiffness=0  SpringStiffnessUnits=N*m/deg  DampingCoefficient=0  DampingCoefficientUnits=N*m/(deg/s)  LowerLimitSpecify=off  LowerLimitBound=-90  LowerLimitBoundUnits=deg  LowerLimitStiffness=1e4  LowerLimitStiffnessUnits=N*m/deg  LowerLimitDamping=10  LowerLimitDampingUnits=N*m/(deg/s)  LowerLimitTransitionRegionWidth=0.1  LowerLimitTransitionRegionWidthUnits=deg  UpperLimitSpecify=off  UpperLimitBound=90  UpperLimitBoundUnits=deg  UpperLimitStiffness=1e4  UpperLimitStiffnessUnits=N*m/deg  UpperLimitDamping=10  UpperLimitDampingUnits=N*m/(deg/s)  UpperLimitTransitionRegionWidth=0.1  UpperLimitTransitionRegionWidthUnits=deg  TorqueActuationMode=ComputedTorque  MotionActuationMode=InputMotion  SensePosition=off  SenseVelocity=off  SenseAcceleration=off  SenseTorqueForce=off  SenseLowerLimitTorqueForce=off  SenseUpperLimitTorqueForce=off
  Revolute3 : sm_lib/Joints/Revolute Joint  JointMode=Normal  CompositeWrenchDir=FollowerOnBase  CompositeWrenchFrame=BaseFrame  SenseConstraintForce=off  SenseConstraintTorque=off  SenseTotalForce=off  SenseTotalTorque=off  PositionTargetSpecify=off  PositionTargetPriority=Low  PositionTargetValue=smiData.RevoluteJoint(4).Rz.Pos  PositionTargetValueUnits=deg  VelocityTargetSpecify=off  VelocityTargetPriority=High  VelocityTargetValue=0  VelocityTargetValueUnits=deg/s  EquilibriumPosition=0  EquilibriumPositionUnits=deg  SpringStiffness=0  SpringStiffnessUnits=N*m/deg  DampingCoefficient=0  DampingCoefficientUnits=N*m/(deg/s)  LowerLimitSpecify=off  LowerLimitBound=-90  LowerLimitBoundUnits=deg  LowerLimitStiffness=1e4  LowerLimitStiffnessUnits=N*m/deg  LowerLimitDamping=10  LowerLimitDampingUnits=N*m/(deg/s)  LowerLimitTransitionRegionWidth=0.1  LowerLimitTransitionRegionWidthUnits=deg  UpperLimitSpecify=off  UpperLimitBound=90  UpperLimitBoundUnits=deg  UpperLimitStiffness=1e4  UpperLimitStiffnessUnits=N*m/deg  UpperLimitDamping=10  UpperLimitDampingUnits=N*m/(deg/s)  UpperLimitTransitionRegionWidth=0.1  UpperLimitTransitionRegionWidthUnits=deg  TorqueActuationMode=ComputedTorque  MotionActuationMode=InputMotion  SensePosition=off  SenseVelocity=off  SenseAcceleration=off  SenseTorqueForce=off  SenseLowerLimitTorqueForce=off  SenseUpperLimitTorqueForce=off
  Revolute4 : sm_lib/Joints/Revolute Joint  JointMode=Normal  CompositeWrenchDir=FollowerOnBase  CompositeWrenchFrame=BaseFrame  SenseConstraintForce=off  SenseConstraintTorque=off  SenseTotalForce=off  SenseTotalTorque=off  PositionTargetSpecify=off  PositionTargetPriority=Low  PositionTargetValue=smiData.RevoluteJoint(5).Rz.Pos  PositionTargetValueUnits=deg  VelocityTargetSpecify=off  VelocityTargetPriority=High  VelocityTargetValue=0  VelocityTargetValueUnits=deg/s  EquilibriumPosition=0  EquilibriumPositionUnits=deg  SpringStiffness=0  SpringStiffnessUnits=N*m/deg  DampingCoefficient=0  DampingCoefficientUnits=N*m/(deg/s)  LowerLimitSpecify=off  LowerLimitBound=-90  LowerLimitBoundUnits=deg  LowerLimitStiffness=1e4  LowerLimitStiffnessUnits=N*m/deg  LowerLimitDamping=10  LowerLimitDampingUnits=N*m/(deg/s)  LowerLimitTransitionRegionWidth=0.1  LowerLimitTransitionRegionWidthUnits=deg  UpperLimitSpecify=off  UpperLimitBound=90  UpperLimitBoundUnits=deg  UpperLimitStiffness=1e4  UpperLimitStiffnessUnits=N*m/deg  UpperLimitDamping=10  UpperLimitDampingUnits=N*m/(deg/s)  UpperLimitTransitionRegionWidth=0.1  UpperLimitTransitionRegionWidthUnits=deg  TorqueActuationMode=ComputedTorque  MotionActuationMode=InputMotion  SensePosition=off  SenseVelocity=off  SenseAcceleration=off  SenseTorqueForce=off  SenseLowerLimitTorqueForce=off  SenseUpperLimitTorqueForce=off
  Revolute5 : sm_lib/Joints/Revolute Joint  JointMode=Normal  CompositeWrenchDir=FollowerOnBase  CompositeWrenchFrame=BaseFrame  SenseConstraintForce=off  SenseConstraintTorque=off  SenseTotalForce=off  SenseTotalTorque=off  PositionTargetSpecify=off  PositionTargetPriority=Low  PositionTargetValue=smiData.RevoluteJoint(6).Rz.Pos  PositionTargetValueUnits=deg  VelocityTargetSpecify=off  VelocityTargetPriority=High  VelocityTargetValue=0  VelocityTargetValueUnits=deg/s  EquilibriumPosition=0  EquilibriumPositionUnits=deg  SpringStiffness=0  SpringStiffnessUnits=N*m/deg  DampingCoefficient=0  DampingCoefficientUnits=N*m/(deg/s)  LowerLimitSpecify=off  LowerLimitBound=-75  LowerLimitBoundUnits=deg  LowerLimitStiffness=1e4  LowerLimitStiffnessUnits=N*m/deg  LowerLimitDamping=10  LowerLimitDampingUnits=N*m/(deg/s)  LowerLimitTransitionRegionWidth=0.1  LowerLimitTransitionRegionWidthUnits=deg  UpperLimitSpecify=off  UpperLimitBound=75  UpperLimitBoundUnits=deg  UpperLimitStiffness=1e4  UpperLimitStiffnessUnits=N*m/deg  UpperLimitDamping=10  UpperLimitDampingUnits=N*m/(deg/s)  UpperLimitTransitionRegionWidth=0.1  UpperLimitTransitionRegionWidthUnits=deg  TorqueActuationMode=ComputedTorque  MotionActuationMode=InputMotion  SensePosition=off  SenseVelocity=off  SenseAcceleration=off  SenseTorqueForce=off  SenseLowerLimitTorqueForce=off  SenseUpperLimitTorqueForce=off
  Scope : Scope
  Simulink-PS Converter{,1..5} (6 alike) : nesl_utility/Simulink-PS Converter  PhysicalDomain=network_engine_domain  SubClassName=ps_input  LeftPortType=input  RightPortType=output  PseudoPeriodic=off  Frequencies=[]  NoiseDistribution=none  NoiseParameters=[]  Unit=1  AffineConversion=off  FilteringAndDerivatives=filter  SimscapeFilterOrder=2  InputFilterTimeConstant=0.001  UdotUserProvided=0
  Solver Configuration : nesl_utility/Solver Configuration  PhysicalDomain=network_engine_domain  SubClassName=solver  LeftPortType=input  RightPortType=generic  Tones=[]  Harmonics=[]  SimulateNoise=off  Profile=off  UseLocalSampling=off  EnableSwitchedLinearOptims=on  FrequencyDomain=off  UseCCode=off  RelTol=0.001  AbsTol=0.001  MinStep=1e-09  ToWorkspace=off  RevertToSquareIcSolve=off  NumHomotopyIterations=100  PhasorMode=off  PhasorModeNumHarmonics=1  ConsistencySolver=NEWTON_XTOL_AFTER_FTOL  IndexReductionMethod=DerivativeReplacement  DoDC=off  ResidualTolerance=1e-09  ConsistencyTolSource=GLOBAL  ConsistencyAbsTol=0.001  ConsistencyRelTol=0.001  ConsistencyTolFactor=0.001  UseLocalSolver=on  LocalSolverChoice=NE_BACKWARD_EULER_ADVANCER  ResolveIndetEquations=on  FunctionEvalNumThread=1  LocalSolverSampleTime=0.001  DoFixedCost=off  MaxNonlinIter=3  MaxModeIter=2  ComputeImpulses=off  ImpulseIterations=2  LinearAlgebra=auto  LinearAlgebraNumThread=0  EquationFormulation=NE_TIME_EF  DelaysMemoryBudget=1024  AutomaticFiltering=on  FilteringTimeConstant=0.001  PartitionStorageMethod=AS_NEEDED  PartitionMemoryBudget=1024  PartitionMethod=ROBUST  MultibodyUseLocalSolver=off  MultibodyLocalSolverChoice=ODE1  MultibodyLocalSolverSampleTime=0.001
  Transform : sm_lib/Frames and Transforms/Rigid Transform  RotationMethod=ArbitraryAxis  FollAlignAxisA=+X  BaseAlignAxisA=+Y  FollAlignAxisB=+Y  BaseAlignAxisB=+Z  RotationStandardAxis=+Z  RotationAngle=smiData.RigidTransform(13).angle  RotationAngleUnits=rad  RotationArbitraryAxis=smiData.RigidTransform(13).axis  RotationSequenceAxes=FollowerAxes  RotationSequence=XYX  RotationSequenceAngles=[0 0 0]  RotationSequenceAnglesUnits=deg  RotationMatrix=[1 0 0; 0 1 0; 0 0 1]  Quaternion=[1 0 0 0]  TranslationMethod=Cartesian  TranslationCartesianOffset=smiData.RigidTransform(13).translation  TranslationCartesianOffsetUnits=m  TranslationStandardAxis=+Z  TranslationStandardOffset=0  TranslationStandardOffsetUnits=m  TranslationROffset=0  TranslationROffsetUnits=m  TranslationThetaOffset=0  TranslationThetaOffsetUnits=deg  TranslationZOffset=0  TranslationZOffsetUnits=m
  World : sm_lib/Frames and Transforms/World Frame
  wires:
  joint6/1 -> Simulink-PS Converter5/1
  joint2/1 -> Simulink-PS Converter1/1
  joint5/1 -> Simulink-PS Converter4/1
  joint3/1 -> Simulink-PS Converter2/1
  joint1/1 -> Scope/1, Simulink-PS Converter/1
  joint4/1 -> Simulink-PS Converter3/1
  connections:
  Transform/LConn1 -- Mechanism Configuration/RConn1 -- Solver Configuration/RConn1 -- World/RConn1
  Base_2_RIGID/RConn1 -- Revolute2/LConn1
  L1_v2_1_RIGID/RConn1 -- Revolute3/LConn1
  L2_v4_1_RIGID/RConn1 -- Revolute5/LConn1
  Simulink-PS Converter1/RConn1 -- Revolute3/LConn2
  Simulink-PS Converter5/RConn1 -- Revolute4/LConn2
  Link3_v2_1_RIGID/RConn1 -- Revolute/LConn1
  Simulink-PS Converter2/RConn1 -- Revolute5/LConn2
  L6_2_RIGID/LConn1 -- Revolute4/RConn1
  Link5_v2_1_RIGID/RConn1 -- Revolute4/LConn1
  Link4_v2_1_RIGID/LConn1 -- Revolute/RConn1
  Link3_v2_1_RIGID/LConn1 -- Revolute5/RConn1
  Link4_v2_1_RIGID/RConn1 -- Revolute1/LConn1
  Base_2_RIGID/LConn1 -- Transform/RConn1
  Simulink-PS Converter4/RConn1 -- Revolute1/LConn2
  Link5_v2_1_RIGID/LConn1 -- Revolute1/RConn1
  L2_v4_1_RIGID/LConn1 -- Revolute3/RConn1
  L1_v2_1_RIGID/LConn1 -- Revolute2/RConn1
  Simulink-PS Converter/RConn1 -- Revolute2/LConn2
  Simulink-PS Converter3/RConn1 -- Revolute/LConn2
